simulink library "engine_S2_lib"  (Simulink 6.6)
libraries: simulink x3, aeroutilslib x1, engine_JetCatP120SE_lib x1
settings Model: Creator=amurch  LastModifiedBy=amurch

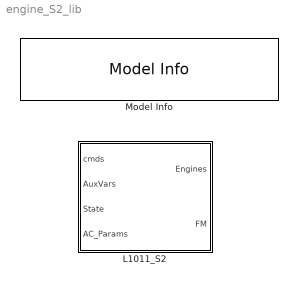
== system engine_S2_lib ==
  L1011_S2 : Subsystem
  Model Info : simulink/Model-Wide Utilities/Model Info  SystemSampleTime=-1  InitialBlockCM=None  BlockCM=None  Frame=on  DisplayStringWithTags=|  HorizontalTextAlignment=Center  LeftAlignmentValue=0.5  SourceBlockDiagram=engine_S2_lib  TagMaxNumber=20
      | L1011 S2 Engine Library
      | 
      | Model Version: %<ModelVersion>
      | Last modifed by %<LastModifiedBy> on %<LastModificationDate>

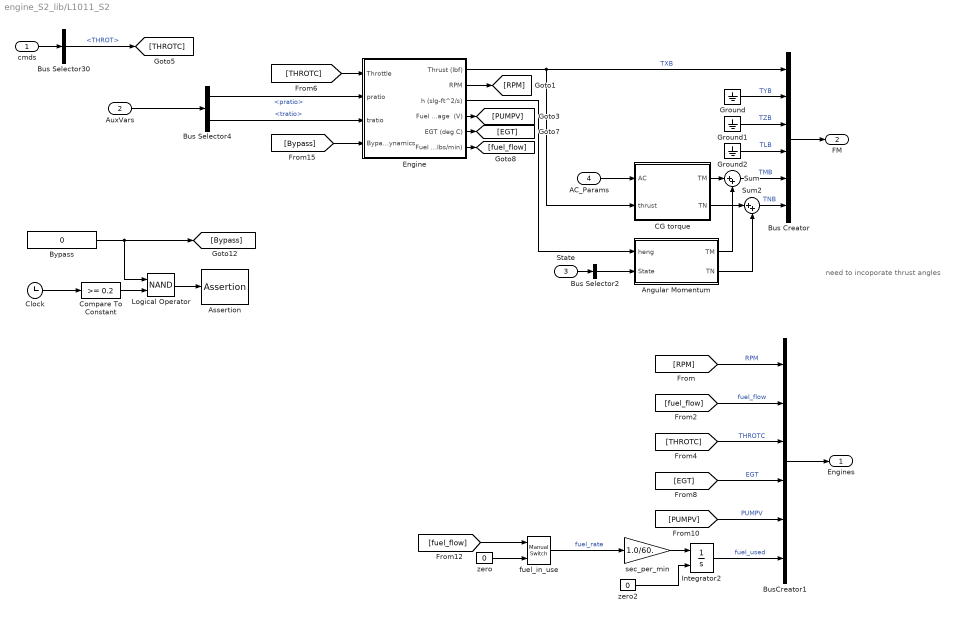
== system engine_S2_lib/L1011_S2 ==
  note: need to incoporate thrust angles
  cmds : Inport
  AuxVars : Inport  Port=2
  State : Inport  Port=3
  AC_Params : Inport  Port=4
  Angular Momentum : Subsystem
  Assertion : Assertion  Enabled=on  AssertionFailFcn=warndlg('Engine dynamics in bypass mode. Run setup.m to reset.','Warning!')
  Bus Creator : BusCreator  Inputs=6
  Bus Selector2 : BusSelector  OutputSignals=pb,qb,rb  OutputAsBus=on
  Bus Selector30 : BusSelector  OutputSignals=THROT
  Bus Selector4 : BusSelector  OutputSignals=pratio,tratio
  BusCreator1 : BusCreator  Inputs=6
  Bypass : Constant  Value=0
  CG torque : Subsystem
  Clock : Clock
      settings: Decimation=10
  Compare To Constant : simulink/Logic and Bit Operations/Compare To Constant  SystemSampleTime=-1  relop=>=  const=0.2  LogicOutDataTypeMode=boolean  ZeroCross=off
  Engine : Subsystem  BlockChoice=Jetcat P120SE
      settings: AttributesFormatString=%<BlockChoice>  TemplateBlock=enginelib/Engine Model  MemberBlocks=AMT-180,AMT-280,Blank,Jetcat P120SE,Jetcat P70
  Ground : Ground
  Ground1 : Ground
  Ground2 : Ground
  Integrator2 : Integrator  InitialConditionSource=external
  Logical Operator : Logic  Operator=NAND  AllPortsSameDT=off  OutDataTypeMode=Boolean
  Sum : Sum  Inputs=|++
  Sum2 : Sum  Inputs=|++
  fuel_in_use : simulink/Signal Routing/Manual Switch  SystemSampleTime=-1  sw=0  action=0  varsize=off
  sec_per_min : Gain  Gain=1.0/60.  SaturateOnIntegerOverflow=on
  zero : Constant  Value=0
  zero2 : Constant  Value=0
  Engines : Outport
  FM : Outport  Port=2  PortDimensions=6
  wires:
  [THROTC] -> Engine/1(Throttle)
  Bus Selector30/1 -> [THROTC]  "<THROT>"
  Bus Creator/1 -> FM/1
  BusCreator1/1 -> Engines/1
  AC_Params/1 -> CG torque/1(AC)
  Bus Selector4/1 -> Engine/2(pratio)  "<pratio>"
  AuxVars/1 -> Bus Selector4/1
  Bus Selector4/2 -> Engine/3(tratio)  "<tratio>"
  Engine/4(Fuel Pump Voltage  (V)) -> [PUMPV]
  Engine/2(RPM) -> [RPM]
  Ground2/1 -> Bus Creator/4  "TLB"
  Ground1/1 -> Bus Creator/3  "TZB"
  Angular Momentum/2(TN) -> Sum2/2
  Angular Momentum/1(TM) -> Sum/2
  CG torque/2(TN) -> Sum2/1
  CG torque/1(TM) -> Sum/1
  Sum/1 -> Bus Creator/5  "TMB"
  Sum2/1 -> Bus Creator/6  "TNB"
  Bus Selector2/1 -> Angular Momentum/2(State)
  State/1 -> Bus Selector2/1
  Engine/1(Thrust (lbf)) -> CG torque/2(thrust), Bus Creator/1  "TXB"
  Ground/1 -> Bus Creator/2  "TYB"
  cmds/1 -> Bus Selector30/1
  Engine/5(EGT (deg C)) -> [EGT]
  Engine/6(Fuel Flow (lbs/min)) -> [fuel_flow]
  sec_per_min/1 -> Integrator2/1
  fuel_in_use/1 -> sec_per_min/1  "fuel_rate"
  zero2/1 -> Integrator2/2
  Engine/3(h (slg-ft^2/s)) -> Angular Momentum/1(heng)
  [RPM] -> BusCreator1/1  "RPM"
  [fuel_flow] -> BusCreator1/2  "fuel_flow"
  [THROTC] -> BusCreator1/3  "THROTC"
  [EGT] -> BusCreator1/4  "EGT"
  [PUMPV] -> BusCreator1/5  "PUMPV"
  Integrator2/1 -> BusCreator1/6  "fuel_used"
  [fuel_flow] -> fuel_in_use/1
  zero/1 -> fuel_in_use/2
  [Bypass] -> Engine/4(BypassDynamics)
  Bypass/1 -> Logical Operator/1, [Bypass]
  Clock/1 -> Compare To Constant/1
  Compare To Constant/1 -> Logical Operator/2
  Logical Operator/1 -> Assertion/1

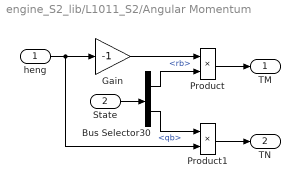
== system engine_S2_lib/L1011_S2/Angular Momentum ==
  heng : Inport
  State : Inport  Port=2
  Bus Selector30 : BusSelector  OutputSignals=rb,qb
  Gain : Gain  Gain=-1  SaturateOnIntegerOverflow=on
  Product : Product  SaturateOnIntegerOverflow=on  InputSameDT=on
  Product1 : Product  SaturateOnIntegerOverflow=on  InputSameDT=on
  TM : Outport
  TN : Outport  Port=2
  wires:
  Gain/1 -> Product/1
  Product1/1 -> TN/1
  Product/1 -> TM/1
  Bus Selector30/2 -> Product1/1  "<qb>"
  Bus Selector30/1 -> Product/2  "<rb>"
  heng/1 -> Gain/1, Product1/2
  State/1 -> Bus Selector30/1

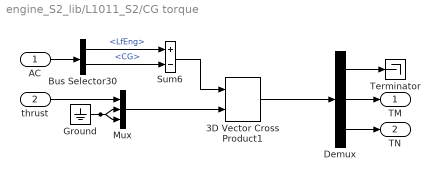
== system engine_S2_lib/L1011_S2/CG torque ==
  AC : Inport
  thrust : Inport  Port=2
  3D Vector Cross Product1 : aeroutilslib/3D Vector Cross Product  SystemSampleTime=-1
  Bus Selector30 : BusSelector  OutputSignals=LfEng,CG
  Demux : Demux  Outputs=3
  Ground : Ground
  Mux : Mux  Inputs=3
  Sum6 : Sum  Inputs=+-  SaturateOnIntegerOverflow=on  InputSameDT=on
  Terminator : Terminator
  TM : Outport
  TN : Outport  Port=2
  wires:
  Bus Selector30/1 -> Sum6/1  "<LfEng>"
  Demux/1 -> Terminator/1
  Demux/3 -> TN/1
  Demux/2 -> TM/1
  3D Vector Cross Product1/1 -> Demux/1
  Sum6/1 -> 3D Vector Cross Product1/1
  Mux/1 -> 3D Vector Cross Product1/2
  Ground/1 -> Mux/3, Mux/2
  thrust/1 -> Mux/1
  Bus Selector30/2 -> Sum6/2  "<CG>"
  AC/1 -> Bus Selector30/1

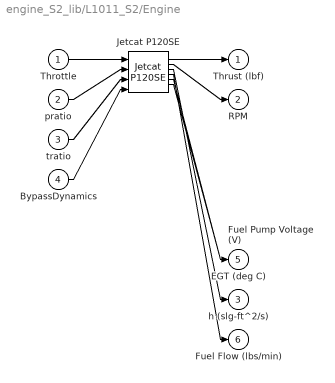
== system engine_S2_lib/L1011_S2/Engine ==
  Throttle : Inport
  pratio : Inport  Port=2
  tratio : Inport  Port=3
  BypassDynamics : Inport  Port=4
  Jetcat P120SE : engine_JetCatP120SE_lib/Jetcat P120SE  SystemSampleTime=-1
  Thrust (lbf) : Outport
  RPM : Outport  Port=2
  h (slg-ft^2/s) : Outport  Port=3
  Fuel Pump Voltage  (V) : Outport  Port=4
  EGT (deg C) : Outport  Port=5
  Fuel Flow (lbs/min) : Outport  Port=6
  wires:
  Throttle/1 -> Jetcat P120SE/1
  pratio/1 -> Jetcat P120SE/2
  tratio/1 -> Jetcat P120SE/3
  BypassDynamics/1 -> Jetcat P120SE/4
  Jetcat P120SE/1 -> Thrust (lbf)/1
  Jetcat P120SE/2 -> RPM/1
  Jetcat P120SE/3 -> h (slg-ft^2/s)/1
  Jetcat P120SE/4 -> Fuel Flow (lbs/min)/1
  Jetcat P120SE/5 -> Fuel Pump Voltage  (V)/1
  Jetcat P120SE/6 -> EGT (deg C)/1
